simulink model "tracking"  (R2021a)
settings: Solver=ode45  StartTime=16665.7001  StopTime=33331.4002  MaxStep=0.1  RelTol=1e-8  AbsTol=1e-8
values from neighbouring files (symbols this model uses):
  spacecraft = struct()    [setup.m]
undefined symbols (not defined in the file or in its folder): actuators, constants, control, orbit
libraries: vrlib x6, library x3
settings Model: SimulationMode=accelerator  Creator=loren  LastModifiedBy=loren
settings SolverCC: ZeroCrossAlgorithm=Adaptive
settings DebuggingCC: IgnoredZcDiagnostic=none

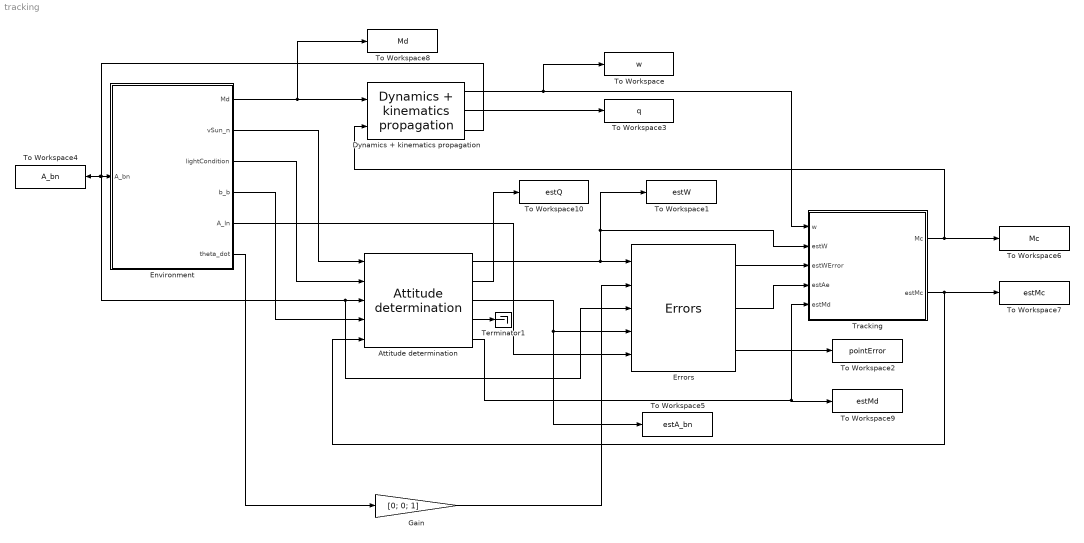
== system tracking ==
  Attitude determination : library/Attitude determination  SystemSampleTime=-1  VariantActivationTime=update diagram  Latency=0  AutoFrameSizeCalculation=off
  Dynamics + kinematics propagation : library/Dynamics + kinematics propagation  SystemSampleTime=-1  VariantActivationTime=update diagram  Latency=0  AutoFrameSizeCalculation=off
  Environment : Subsystem  AncestorBlock=library/Environment
  Errors : library/Errors  SystemSampleTime=-1  VariantActivationTime=update diagram  Latency=0  AutoFrameSizeCalculation=off
  Gain : Gain  Gain=[0; 0; 1]
  Terminator1 : Terminator
  To Workspace : ToWorkspace  VariableName=w  SampleTime=-1
  To Workspace1 : ToWorkspace  VariableName=estW  SampleTime=-1
  To Workspace10 : ToWorkspace  VariableName=estQ  SampleTime=-1
  To Workspace2 : ToWorkspace  VariableName=pointError  SampleTime=-1
  To Workspace3 : ToWorkspace  VariableName=q  SampleTime=-1
  To Workspace4 : ToWorkspace  VariableName=A_bn  SampleTime=-1
  To Workspace5 : ToWorkspace  VariableName=estA_bn  SampleTime=-1
  To Workspace6 : ToWorkspace  VariableName=Mc  SampleTime=-1
  To Workspace7 : ToWorkspace  VariableName=estMc  SampleTime=-1
  To Workspace8 : ToWorkspace  VariableName=Md  SampleTime=-1
  To Workspace9 : ToWorkspace  VariableName=estMd  SampleTime=-1
  Tracking : Subsystem  AncestorBlock=library/Tracking
  wires:
  Environment/5(A_ln) -> Errors/5
  Gain/1 -> Errors/2
  Dynamics + kinematics propagation/1 -> Tracking/1(w), To Workspace/1
  Errors/3 -> To Workspace2/1
  Environment/1(Md) -> To Workspace8/1, Dynamics + kinematics propagation/1
  Errors/1 -> Tracking/3(estWError)
  Tracking/2(estMc) -> Attitude determination/5, To Workspace7/1
  Errors/2 -> Tracking/4(estAe)
  Dynamics + kinematics propagation/2 -> To Workspace3/1
  Attitude determination/1 -> Tracking/2(estW), To Workspace1/1, Errors/1
  Environment/4(b_b) -> Attitude determination/4
  Attitude determination/2 -> To Workspace10/1
  Environment/6(theta_dot) -> Gain/1
  Dynamics + kinematics propagation/3 -> To Workspace4/1, Environment/1(A_bn), Errors/3, Attitude determination/3
  Environment/2(vSun_n) -> Attitude determination/1
  Tracking/1(Mc) -> Dynamics + kinematics propagation/2, To Workspace6/1
  Attitude determination/5 -> Tracking/5(estMd), To Workspace9/1
  Attitude determination/3 -> To Workspace5/1, Errors/4
  Environment/3(lightCondition) -> Attitude determination/2
  Attitude determination/4 -> Terminator1/1

== system tracking/Environment ==
  A_bn : Inport
  Disturbances : Subsystem
  Orbit propagator : Subsystem
  Md : Outport
  vSun_n : Outport  Port=2
  lightCondition : Outport  Port=3
  b_b : Outport  Port=4
  A_ln : Outport  Port=5
  theta_dot : Outport  Port=6
  wires:
  Orbit propagator/4(A_ln) -> A_ln/1
  Orbit propagator/5(theta_dot) -> theta_dot/1
  Disturbances/4(b_b) -> b_b/1
  Disturbances/3(lightCondition) -> lightCondition/1
  Disturbances/2(vSun_n) -> vSun_n/1
  Disturbances/1(Md) -> Md/1
  Orbit propagator/3(A_bl) -> Disturbances/4(A_bl)
  Orbit propagator/2(vvSc_n) -> Disturbances/3(vvSc_n)
  Orbit propagator/1(rrSc_n) -> Disturbances/2(rrSc_n)
  A_bn/1 -> Disturbances/1(A_bn), Orbit propagator/1(A_bn)

== system tracking/Tracking ==
  w : Inport
  estW : Inport  Port=2
  estWError : Inport  Port=3
  estAe : Inport  Port=4
  estMd : Inport  Port=5
  Ideal control law : Subsystem
  Reaction wheels : Subsystem  AncestorBlock=library/Reaction wheels
  Mc : Outport
  estMc : Outport  Port=2
  wires:
  Reaction wheels/2(estMc_RW) -> estMc/1
  Reaction wheels/1(Mc_RW) -> Mc/1
  estMd/1 -> Ideal control law/4(estMd)
  estAe/1 -> Ideal control law/3(estAe)
  estWError/1 -> Ideal control law/2(estWError)
  estW/1 -> Ideal control law/1(estW), Reaction wheels/3(estW)
  Ideal control law/1(Mc_id) -> Reaction wheels/1(targetMc)
  w/1 -> Reaction wheels/2(w)

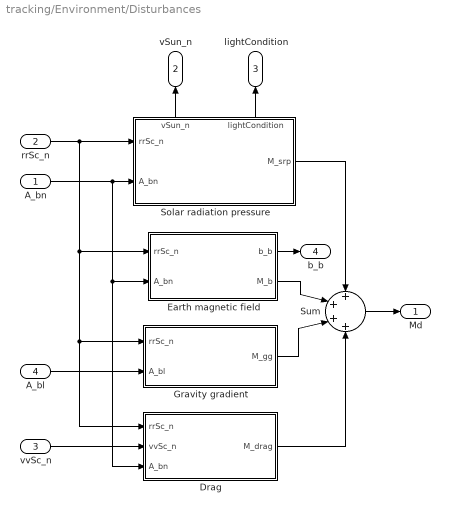
== system tracking/Environment/Disturbances ==
  A_bn : Inport
  rrSc_n : Inport  Port=2
  vvSc_n : Inport  Port=3
  A_bl : Inport  Port=4
  Drag : Subsystem
  Earth magnetic field : Subsystem
  Gravity gradient : Subsystem
  Solar radiation pressure : Subsystem
      settings: PortSchema="{\"entries\":[{\"content\":{\"sides\":[{\"content\":{\"connectorIds\":[\"In1\",\"In2\"]},\"type\":\"ConnectorPlacement.EquallySpacedRectSide\",\"uuid\":\"1c58e148-737e-4c26-8467-bf4a1427bac3\"},{\"content\":{\"connectorIds\":[\"Out1\"],\"side\":\"RIGHT\"},\"type\":\"ConnectorPlacement.EquallySpacedRectSide\",\"uuid\":\"1132a1c1-392d-4550-8b40-4ae647f3a6c1\"},{\"content\":{\"connectorIds\":[\"Out2\",\"Out3\"],\"side\":\"TOP\"},\"type\":\"ConnectorPlacement.EquallySpacedRectSide\",\"uuid\":\"8cec875a-7b2b-408d-843f-f50e353248f2\"},{\"content\":{\"connectorIds\":[],\"side\":\"HIDDEN\"},\"type\":\"ConnectorPlacement.EquallySpacedRectSide\",\"uuid\":\"95559ba3-4215-4144-a5e7-008848b1ca72\"}]},\"type\":\"ConnectorPlacement.EquallySpacedConnector\",\"uuid\":\"cb15f690-b6d7-424c-84c7-df23a46a4e4f\"}],\"packageUris\":[\"http://schema.mathworks.com/mf0/Connector/R2020b\"],\"version\":\"1.0\"}"
  Sum : Sum  Inputs=++++
  Md : Outport
  vSun_n : Outport  Port=2
  lightCondition : Outport  Port=3
  b_b : Outport  Port=4
  wires:
  Earth magnetic field/1(b_b) -> b_b/1
  Solar radiation pressure/3(lightCondition) -> lightCondition/1
  Solar radiation pressure/2(vSun_n) -> vSun_n/1
  A_bl/1 -> Gravity gradient/2(A_bl)
  Sum/1 -> Md/1
  Earth magnetic field/2(M_b) -> Sum/2
  Drag/1(M_drag) -> Sum/4
  Gravity gradient/1(M_gg) -> Sum/3
  rrSc_n/1 -> Solar radiation pressure/1(rrSc_n), Earth magnetic field/1(rrSc_n), Drag/1(rrSc_n), Gravity gradient/1(rrSc_n)
  vvSc_n/1 -> Drag/2(vvSc_n)
  A_bn/1 -> Earth magnetic field/2(A_bn), Drag/3(A_bn), Solar radiation pressure/2(A_bn)
  Solar radiation pressure/1(M_srp) -> Sum/1

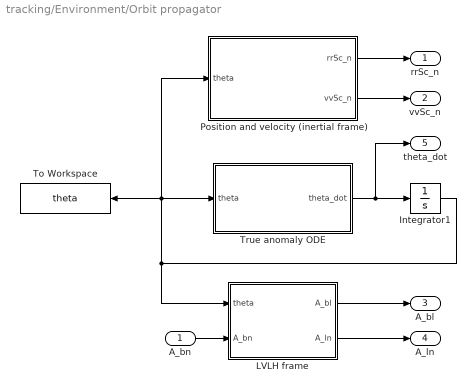
== system tracking/Environment/Orbit propagator ==
  A_bn : Inport
  Integrator1 : Integrator  InitialCondition=orbit.theta0
  LVLH frame : Subsystem
  Position and velocity (inertial frame) : Subsystem
  To Workspace : ToWorkspace  VariableName=theta  SampleTime=-1
  True anomaly ODE : Subsystem
  rrSc_n : Outport
  vvSc_n : Outport  Port=2
  A_bl : Outport  Port=3
  A_ln : Outport  Port=4
  theta_dot : Outport  Port=5
  wires:
  LVLH frame/2(A_ln) -> A_ln/1
  A_bn/1 -> LVLH frame/2(A_bn)
  LVLH frame/1(A_bl) -> A_bl/1
  Position and velocity (inertial frame)/2(vvSc_n) -> vvSc_n/1
  Position and velocity (inertial frame)/1(rrSc_n) -> rrSc_n/1
  Integrator1/1 -> To Workspace/1, Position and velocity (inertial frame)/1(theta), True anomaly ODE/1(theta), LVLH frame/1(theta)
  True anomaly ODE/1(theta_dot) -> theta_dot/1, Integrator1/1

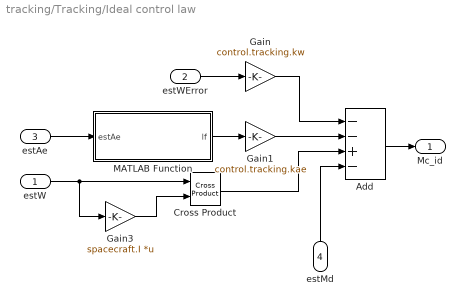
== system tracking/Tracking/Ideal control law ==
  estW : Inport
  estWError : Inport  Port=2
  estAe : Inport  Port=3
  estMd : Inport  Port=4
  Add : Sum  Inputs=--+-
  Cross Product : vrlib/Utilities/Cross Product
  Gain : Gain  Gain=control.tracking.kw
  Gain1 : Gain  Gain=control.tracking.kae
  Gain3 : Gain  Gain=spacecraft.I  Multiplication=Matrix(K*u) (u vector)
  MATLAB Function : MATLAB Function  TreatAsAtomicUnit=on
  Mc_id : Outport
  wires:
  Cross Product/1 -> Add/3
  estW/1 -> Cross Product/1, Gain3/1
  estWError/1 -> Gain/1
  Gain1/1 -> Add/2
  estMd/1 -> Add/4
  Gain3/1 -> Cross Product/2
  Gain/1 -> Add/1
  estAe/1 -> MATLAB Function/1(estAe)
  MATLAB Function/1(lf) -> Gain1/1
  Add/1 -> Mc_id/1

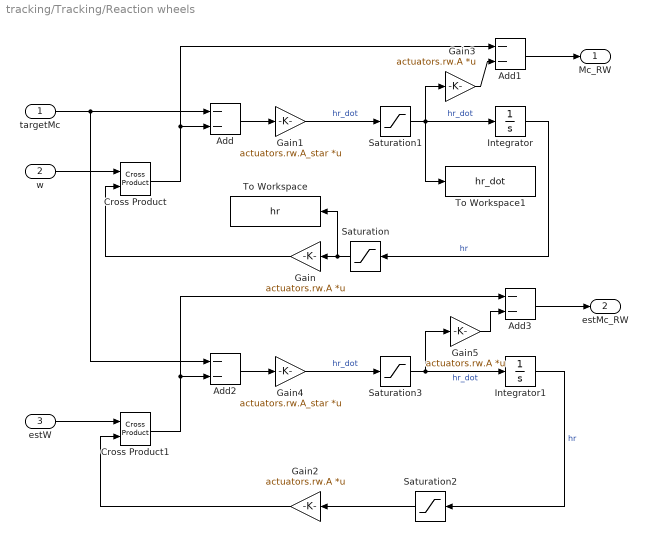
== system tracking/Tracking/Reaction wheels ==
  targetMc : Inport
  w : Inport  Port=2
  estW : Inport  Port=3
  Add{,1..3} (4 alike) : Sum  Inputs=--
  Cross Product : vrlib/Utilities/Cross Product
  Cross Product1 : vrlib/Utilities/Cross Product
  Gain{,2..3,5} (4 alike) : Gain  Gain=actuators.rw.A  Multiplication=Matrix(K*u) (u vector)
  Gain1 : Gain  Gain=actuators.rw.A_star  Multiplication=Matrix(K*u) (u vector)
  Gain4 : Gain  Gain=actuators.rw.A_star  Multiplication=Matrix(K*u) (u vector)
  Integrator : Integrator  InitialCondition=actuators.rw.hr0
  Integrator1 : Integrator  InitialCondition=actuators.rw.hr0
  Saturation : Saturate  UpperLimit=actuators.rw.h_max  LowerLimit=-actuators.rw.h_max
  Saturation1 : Saturate  UpperLimit=actuators.rw.hdot_max  LowerLimit=-actuators.rw.hdot_max
  Saturation2 : Saturate  UpperLimit=actuators.rw.h_max  LowerLimit=-actuators.rw.h_max
  Saturation3 : Saturate  UpperLimit=actuators.rw.hdot_max  LowerLimit=-actuators.rw.hdot_max
  To Workspace : ToWorkspace  VariableName=hr  SampleTime=-1
  To Workspace1 : ToWorkspace  VariableName=hr_dot  SampleTime=-1
  Mc_RW : Outport
  estMc_RW : Outport  Port=2
  wires:
  w/1 -> Cross Product/1
  Gain/1 -> Cross Product/2
  Cross Product/1 -> Add/2, Add1/1
  Gain1/1 -> Saturation1/1  "hr_dot"
  Integrator/1 -> Saturation/1  "hr"
  Saturation/1 -> To Workspace/1, Gain/1
  Add1/1 -> Mc_RW/1
  Add/1 -> Gain1/1
  Gain3/1 -> Add1/2
  Saturation1/1 -> To Workspace1/1, Gain3/1, Integrator/1  "hr_dot"
  Gain5/1 -> Add3/2
  Add3/1 -> estMc_RW/1
  Add2/1 -> Gain4/1
  Saturation3/1 -> Integrator1/1, Gain5/1  "hr_dot"
  Cross Product1/1 -> Add2/2, Add3/1
  Integrator1/1 -> Saturation2/1  "hr"
  estW/1 -> Cross Product1/1
  targetMc/1 -> Add2/1, Add/1
  Saturation2/1 -> Gain2/1
  Gain2/1 -> Cross Product1/2
  Gain4/1 -> Saturation3/1  "hr_dot"

== system tracking/Environment/Disturbances/Drag ==
  rrSc_n : Inport
  vvSc_n : Inport  Port=2
  A_bn : Inport  Port=3
  Constant : Constant  Value=constants.rho
  MATLAB Function : MATLAB Function  TreatAsAtomicUnit=on
  M_drag : Outport
  wires:
  Constant/1 -> MATLAB Function/4(rho)
  A_bn/1 -> MATLAB Function/3(A_bn)
  vvSc_n/1 -> MATLAB Function/2(vvSc_n)
  MATLAB Function/1(mDrag) -> M_drag/1
  rrSc_n/1 -> MATLAB Function/1(rrSc_n)

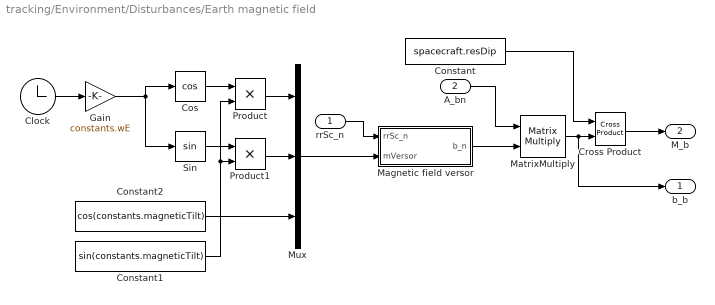
== system tracking/Environment/Disturbances/Earth magnetic field ==
  rrSc_n : Inport
  A_bn : Inport  Port=2
  Clock : Clock
  Constant : Constant  Value=spacecraft.resDip
  Constant1 : Constant  Value=sin(constants.magneticTilt)
  Constant2 : Constant  Value=cos(constants.magneticTilt)
  Cos : Trigonometry  Operator=cos
  Cross Product : vrlib/Utilities/Cross Product
  Gain : Gain  Gain=constants.wE
  Magnetic field versor : Subsystem
  MatrixMultiply : Product  Multiplication=Matrix(*)
  Mux : Mux  Inputs=3
  Product : Product
  Product1 : Product
  Sin : Trigonometry
  b_b : Outport
  M_b : Outport  Port=2
  wires:
  Cross Product/1 -> M_b/1
  MatrixMultiply/1 -> Cross Product/2, b_b/1
  Magnetic field versor/1(b_n) -> MatrixMultiply/2
  Mux/1 -> Magnetic field versor/2(mVersor)
  rrSc_n/1 -> Magnetic field versor/1(rrSc_n)
  A_bn/1 -> MatrixMultiply/1
  Constant1/1 -> Product1/2, Product/2
  Product1/1 -> Mux/2
  Product/1 -> Mux/1
  Cos/1 -> Product/1
  Sin/1 -> Product1/1
  Constant2/1 -> Mux/3
  Gain/1 -> Cos/1, Sin/1
  Constant/1 -> Cross Product/1
  Clock/1 -> Gain/1

== system tracking/Environment/Disturbances/Gravity gradient ==
  rrSc_n : Inport
  A_bl : Inport  Port=2
  Constant : Constant  Value=[1 0 0]
  Gravity gradient : Subsystem
  MatrixMultiply : Product  Multiplication=Matrix(*)
  M_gg : Outport
  wires:
  rrSc_n/1 -> Gravity gradient/1(rrSc_n)
  Gravity gradient/1(M_gg) -> M_gg/1
  A_bl/1 -> MatrixMultiply/1
  MatrixMultiply/1 -> Gravity gradient/2(c)  "c"
  Constant/1 -> MatrixMultiply/2

== system tracking/Environment/Disturbances/Solar radiation pressure ==
  note: Determine whether the s/c is in sunlight or not
  rrSc_n : Inport
  A_bn : Inport  Port=2
  If : If  IfExpression=u1 == 1
  Merge : Merge
  SRP: active : Subsystem  TreatAsAtomicUnit=on
  SRP: non-active : Subsystem  TreatAsAtomicUnit=on
  Shadow cone of the Earth : Subsystem
  Sun position in the Earth inertial frame : Subsystem
  M_srp : Outport
  vSun_n : Outport  Port=2
  lightCondition : Outport  Port=3
  wires:
  A_bn/1 -> SRP: active/3(A_bn)
  SRP: active/2(vSun_n) -> vSun_n/1
  Sun position in the Earth inertial frame/1(rrSun_n) -> Shadow cone of the Earth/2(rrSun_n), SRP: active/2(rrSun_n)
  SRP: active/1(mSRP) -> Merge/1
  Merge/1 -> M_srp/1
  rrSc_n/1 -> Shadow cone of the Earth/1(rrSc_n), SRP: active/1(rrSc_n)
  SRP: non-active/1(mSRP) -> Merge/2
  If/1 -> SRP: active/Action
  If/2 -> SRP: non-active/Action
  Shadow cone of the Earth/1(lightCondition) -> If/1, lightCondition/1

== system tracking/Environment/Orbit propagator/LVLH frame ==
  theta : Inport
  A_bn : Inport  Port=2
  LVLH to inclined orbit frame : Subsystem
  Product : Product  Multiplication=Matrix(*)
  Product1 : Product  Multiplication=Matrix(*)
  R1(i) : Constant  Value=[1 0 0; 0 cos(orbit.i) sin(orbit.i); 0 -sin(orbit.i) cos(orbit.i)];
  Transpose : Math  Operator=transpose  SaturateOnIntegerOverflow=on
  A_bl : Outport
  A_ln : Outport  Port=2
  wires:
  LVLH to inclined orbit frame/1(A_li) -> Product/1
  theta/1 -> LVLH to inclined orbit frame/1(theta)
  R1(i)/1 -> Product/2
  Product1/1 -> A_bl/1  "A_bl"
  A_bn/1 -> Product1/1
  Product/1 -> Transpose/1, A_ln/1
  Transpose/1 -> Product1/2  "A_nl"

== system tracking/Environment/Orbit propagator/Position and velocity (inertial frame) ==
  theta : Inport
  Matrix Multiply : Product  Multiplication=Matrix(*)
  Matrix Multiply1 : Product  Multiplication=Matrix(*)
  Position and velocity (perifocal frame) : Subsystem
  R1(i) : Constant  Value=[1 0 0; 0 cos(orbit.i) sin(orbit.i); 0 -sin(orbit.i) cos(orbit.i)];
  R3(OM) : Constant  Value=[cos(orbit.OM), sin(orbit.OM), 0; -sin(orbit.OM), cos(orbit.OM), 0; 0, 0, 1]
  R3(om) : Constant  Value=[cos(orbit.om), sin(orbit.om), 0; -sin(orbit.om), cos(orbit.om), 0; 0, 0, 1]
  Rotation matrix (perifocal-inertial) : Product  Inputs=3  Multiplication=Matrix(*)
  Transpose : Math  Operator=transpose  SaturateOnIntegerOverflow=on
  rrSc_n : Outport
  vvSc_n : Outport  Port=2
  wires:
  theta/1 -> Position and velocity (perifocal frame)/1(theta)
  Position and velocity (perifocal frame)/1(rrSc_pf) -> Matrix Multiply/2
  R3(OM)/1 -> Rotation matrix (perifocal-inertial)/3
  Transpose/1 -> Matrix Multiply/1, Matrix Multiply1/1
  Rotation matrix (perifocal-inertial)/1 -> Transpose/1
  R1(i)/1 -> Rotation matrix (perifocal-inertial)/2
  R3(om)/1 -> Rotation matrix (perifocal-inertial)/1
  Matrix Multiply1/1 -> vvSc_n/1
  Position and velocity (perifocal frame)/2(vvSc_pf) -> Matrix Multiply1/2
  Matrix Multiply/1 -> rrSc_n/1

== system tracking/Environment/Orbit propagator/True anomaly ODE ==
  theta : Inport
  Add : Sum
  Constant1 : Constant
  Cos : Trigonometry  Operator=cos
  Gain : Gain  Gain=sqrt(constants.mu/orbit.a^3)
  Gain1 : Gain  Gain=(1 - orbit.e^2)^(-3/2)
  Gain2 : Gain  Gain=orbit.e
  Power : Math  Operator=square  SaturateOnIntegerOverflow=on
  theta_dot : Outport
  wires:
  Gain1/1 -> theta_dot/1
  Gain/1 -> Gain1/1
  Power/1 -> Gain/1
  Add/1 -> Power/1
  Gain2/1 -> Add/2
  Cos/1 -> Gain2/1
  Constant1/1 -> Add/1
  theta/1 -> Cos/1

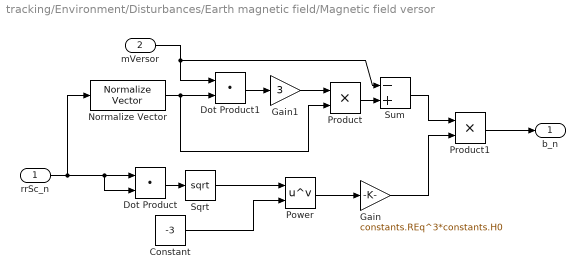
== system tracking/Environment/Disturbances/Earth magnetic field/Magnetic field versor ==
  rrSc_n : Inport
  mVersor : Inport  Port=2
  Constant : Constant  Value=-3
  Dot Product : DotProduct  InputSameDT=on  OutDataTypeStr=Inherit: Inherit via internal rule
  Dot Product1 : DotProduct  InputSameDT=on  OutDataTypeStr=Inherit: Inherit via internal rule
  Gain : Gain  Gain=constants.REq^3*constants.H0
  Gain1 : Gain  Gain=3
  Normalize Vector : vrlib/Utilities/Normalize Vector  maxzero=0
  Power : Math  Operator=pow  SaturateOnIntegerOverflow=on
  Product : Product
  Product1 : Product
  Sqrt : Sqrt  SaturateOnIntegerOverflow=on
  Sum : Sum  Inputs=-+
  b_n : Outport
  wires:
  Product1/1 -> b_n/1
  Gain/1 -> Product1/2
  Sum/1 -> Product1/1
  Product/1 -> Sum/2
  Gain1/1 -> Product/1
  Dot Product1/1 -> Gain1/1
  mVersor/1 -> Dot Product1/1, Sum/1
  Normalize Vector/1 -> Dot Product1/2, Product/2
  Power/1 -> Gain/1
  Sqrt/1 -> Power/1
  Dot Product/1 -> Sqrt/1
  Constant/1 -> Power/2
  rrSc_n/1 -> Dot Product/1, Dot Product/2, Normalize Vector/1

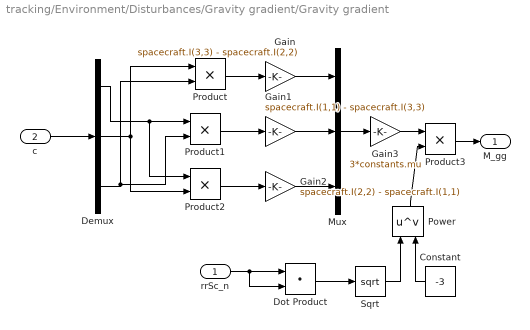
== system tracking/Environment/Disturbances/Gravity gradient/Gravity gradient ==
  rrSc_n : Inport
  c : Inport  Port=2
  Constant : Constant  Value=-3
  Demux : Demux  Outputs=3
  Dot Product : DotProduct  InputSameDT=on  OutDataTypeStr=Inherit: Inherit via internal rule
  Gain : Gain  Gain=spacecraft.I(3,3) - spacecraft.I(2,2)
  Gain1 : Gain  Gain=spacecraft.I(1,1) - spacecraft.I(3,3)
  Gain2 : Gain  Gain=spacecraft.I(2,2) - spacecraft.I(1,1)
  Gain3 : Gain  Gain=3*constants.mu
  Mux : Mux  Inputs=3
  Power : Math  Operator=pow  SaturateOnIntegerOverflow=on
  Product{,1..3} (4 alike) : Product
  Sqrt : Sqrt  SaturateOnIntegerOverflow=on
  M_gg : Outport
  wires:
  Constant/1 -> Power/2
  Power/1 -> Product3/2
  Sqrt/1 -> Power/1
  Dot Product/1 -> Sqrt/1
  rrSc_n/1 -> Dot Product/1, Dot Product/2
  Product3/1 -> M_gg/1
  Gain3/1 -> Product3/1
  Mux/1 -> Gain3/1
  Gain/1 -> Mux/1
  Gain1/1 -> Mux/2
  Gain2/1 -> Mux/3
  Demux/1 -> Product1/1, Product2/1
  Demux/3 -> Product/2, Product1/2
  Demux/2 -> Product/1, Product2/2
  Product2/1 -> Gain2/1
  Product1/1 -> Gain1/1
  Product/1 -> Gain/1
  c/1 -> Demux/1

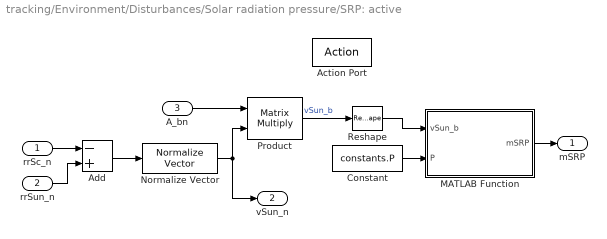
== system tracking/Environment/Disturbances/Solar radiation pressure/SRP: active ==
  rrSc_n : Inport
  rrSun_n : Inport  Port=2
  A_bn : Inport  Port=3
  Action Port : ActionPort  ActionPortLabel=if(u1 == 1)
  Add : Sum  Inputs=-+
  Constant : Constant  Value=constants.P
  MATLAB Function : MATLAB Function  TreatAsAtomicUnit=on
  Normalize Vector : vrlib/Utilities/Normalize Vector  maxzero=0
  Product : Product  Multiplication=Matrix(*)
  Reshape : Reshape  OutputDimensionality=Column vector (2-D)
  mSRP : Outport
  vSun_n : Outport  Port=2
  wires:
  Reshape/1 -> MATLAB Function/1(vSun_b)
  Constant/1 -> MATLAB Function/2(P)
  rrSc_n/1 -> Add/1
  MATLAB Function/1(mSRP) -> mSRP/1
  Add/1 -> Normalize Vector/1
  Normalize Vector/1 -> Product/2, vSun_n/1
  Product/1 -> Reshape/1  "vSun_b"
  rrSun_n/1 -> Add/2
  A_bn/1 -> Product/1

== system tracking/Environment/Disturbances/Solar radiation pressure/SRP: non-active ==
  Action Port : ActionPort  ActionPortLabel=else
  Constant1 : Constant  Value=[0;0;0]
  mSRP : Outport
  wires:
  Constant1/1 -> mSRP/1

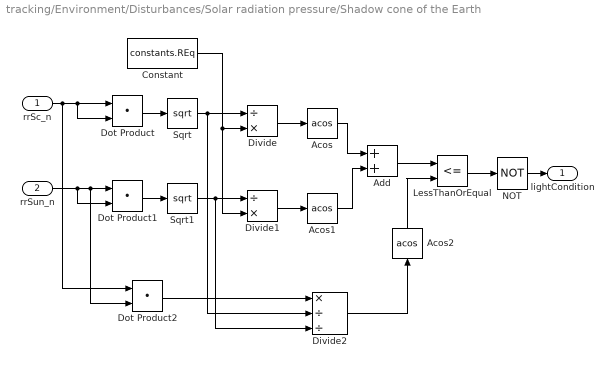
== system tracking/Environment/Disturbances/Solar radiation pressure/Shadow cone of the Earth ==
  rrSc_n : Inport
  rrSun_n : Inport  Port=2
  Acos : Trigonometry  Operator=acos
  Acos1 : Trigonometry  Operator=acos
  Acos2 : Trigonometry  Operator=acos
  Add : Sum
  Constant : Constant  Value=constants.REq
  Divide : Product  Inputs=/*
  Divide1 : Product  Inputs=/*
  Divide2 : Product  Inputs=*//
  Dot Product : DotProduct  InputSameDT=on  OutDataTypeStr=Inherit: Inherit via internal rule
  Dot Product1 : DotProduct  InputSameDT=on  OutDataTypeStr=Inherit: Inherit via internal rule
  Dot Product2 : DotProduct  InputSameDT=on  OutDataTypeStr=Inherit: Inherit via internal rule
  LessThanOrEqual : RelationalOperator  Operator=<=  OutDataTypeStr=boolean  RndMeth=Simplest
  NOT : Logic  Operator=NOT  IconShape=distinctive  AllPortsSameDT=off  OutDataTypeStr=boolean
  Sqrt : Sqrt  SaturateOnIntegerOverflow=on
  Sqrt1 : Sqrt  SaturateOnIntegerOverflow=on
  lightCondition : Outport
  wires:
  Acos2/1 -> LessThanOrEqual/2
  NOT/1 -> lightCondition/1
  LessThanOrEqual/1 -> NOT/1
  Divide2/1 -> Acos2/1
  Add/1 -> LessThanOrEqual/1
  Acos1/1 -> Add/2
  Acos/1 -> Add/1
  Dot Product2/1 -> Divide2/1
  Divide1/1 -> Acos1/1
  Divide/1 -> Acos/1
  Constant/1 -> Divide/2, Divide1/2
  Sqrt1/1 -> Divide1/1, Divide2/3
  Sqrt/1 -> Divide/1, Divide2/2
  rrSun_n/1 -> Dot Product1/1, Dot Product2/2, Dot Product1/2
  Dot Product1/1 -> Sqrt1/1
  Dot Product/1 -> Sqrt/1
  rrSc_n/1 -> Dot Product/1, Dot Product/2, Dot Product2/1

== system tracking/Environment/Disturbances/Solar radiation pressure/Sun position in the Earth inertial frame ==
  Clock : Clock
  Cos : Trigonometry  Operator=cos
  Gain : Gain  Gain=constants.nSun
  Gain1 : Gain  Gain=cos(constants.oblAngle)
  Gain2 : Gain  Gain=sin(constants.oblAngle)
  Gain3 : Gain  Gain=1*constants.AU
  Mux : Mux  Inputs=3
  Sin1 : Trigonometry
  rrSun_n : Outport
  wires:
  Gain3/1 -> rrSun_n/1
  Cos/1 -> Mux/1
  Sin1/1 -> Gain1/1, Gain2/1
  Mux/1 -> Gain3/1
  Gain1/1 -> Mux/2
  Gain/1 -> Cos/1, Sin1/1
  Clock/1 -> Gain/1
  Gain2/1 -> Mux/3

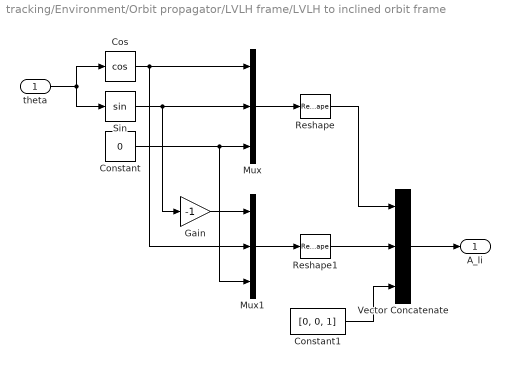
== system tracking/Environment/Orbit propagator/LVLH frame/LVLH to inclined orbit frame ==
  theta : Inport
  Constant : Constant  Value=0
  Constant1 : Constant  Value=[0, 0, 1]  VectorParams1D=off
  Cos : Trigonometry  Operator=cos
  Gain : Gain  Gain=-1
  Mux : Mux  Inputs=3
  Mux1 : Mux  Inputs=3
  Reshape : Reshape  OutputDimensionality=Row vector (2-D)
  Reshape1 : Reshape  OutputDimensionality=Row vector (2-D)
  Sin : Trigonometry
  Vector Concatenate : Concatenate  NumInputs=3  Mode=Multidimensional array
  A_li : Outport
  wires:
  Reshape1/1 -> Vector Concatenate/2
  Reshape/1 -> Vector Concatenate/1
  Vector Concatenate/1 -> A_li/1
  Mux1/1 -> Reshape1/1
  Constant1/1 -> Vector Concatenate/3
  Mux/1 -> Reshape/1
  Gain/1 -> Mux1/1
  Constant/1 -> Mux/3, Mux1/3
  Sin/1 -> Mux/2, Gain/1
  Cos/1 -> Mux/1, Mux1/2
  theta/1 -> Cos/1, Sin/1

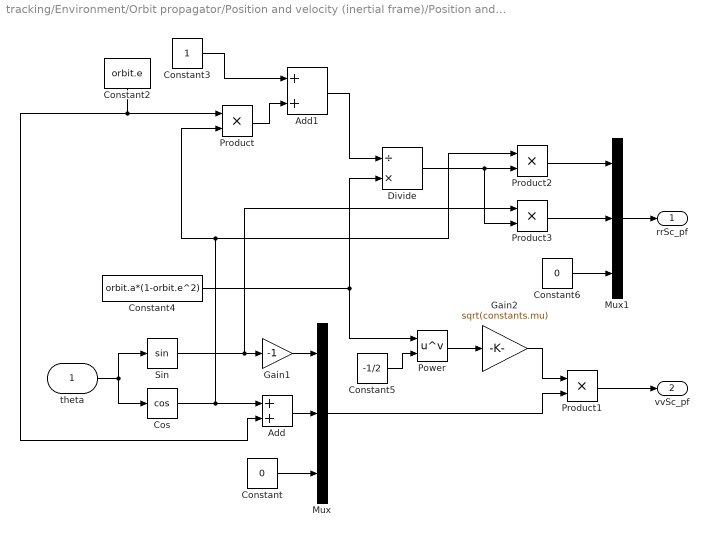
== system tracking/Environment/Orbit propagator/Position and velocity (inertial frame)/Position and velocity (perifocal frame) ==
  theta : Inport
  Add : Sum
  Add1 : Sum
  Constant : Constant  Value=0
  Constant2 : Constant  Value=orbit.e
  Constant3 : Constant
  Constant4 : Constant  Value=orbit.a*(1-orbit.e^2)
  Constant5 : Constant  Value=-1/2
  Constant6 : Constant  Value=0
  Cos : Trigonometry  Operator=cos
  Divide : Product  Inputs=/*
  Gain1 : Gain  Gain=-1
  Gain2 : Gain  Gain=sqrt(constants.mu)
  Mux : Mux  Inputs=3
  Mux1 : Mux  Inputs=3
  Power : Math  Operator=pow  SaturateOnIntegerOverflow=on
  Product{,1..3} (4 alike) : Product
  Sin : Trigonometry
  rrSc_pf : Outport
  vvSc_pf : Outport  Port=2
  wires:
  Mux1/1 -> rrSc_pf/1
  Constant6/1 -> Mux1/3
  Product3/1 -> Mux1/2
  Product2/1 -> Mux1/1
  Divide/1 -> Product2/2, Product3/2
  Gain2/1 -> Product1/1
  Power/1 -> Gain2/1
  Constant5/1 -> Power/2
  Constant4/1 -> Power/1, Divide/2
  Add1/1 -> Divide/1
  Product/1 -> Add1/2
  Constant2/1 -> Product/1, Add/2
  Constant3/1 -> Add1/1
  Product1/1 -> vvSc_pf/1
  Constant/1 -> Mux/3
  Add/1 -> Mux/2
  Gain1/1 -> Mux/1
  Cos/1 -> Add/1, Product/2, Product2/1
  Sin/1 -> Gain1/1, Product3/1
  Mux/1 -> Product1/2
  theta/1 -> Sin/1, Cos/1

== matlab function tracking/Environment/Disturbances/Solar radiation pressure/SRP: active/MATLAB Function ==
  data: vSun_b input; P input; mSRP output; surfaces parameter
function mSRP = srp(vSun_b, P, surfaces)

rSurf = surfaces.rSurf;
n = surfaces.n;
A = surfaces.A;
rhoS = surfaces.rhoS;
rhoD = surfaces.rhoD;

% Preallocation
mSRP = zeros(3,1);

% Loop on the number of surfaces
for k = 1:size(rSurf,1)
    % Extraction of the normal vector
    n_b = n(:,k);
    s_dot = dot(vSun_b, n_b);
    if s_dot > 0
        rhoS_temp = rhoS(k);
        Fsrp_i = - P*A(k)*s_dot.*((1-rhoS_temp).*vSun_b +...
            (2*rhoS_temp*s_dot + 2/3*rhoD(k)).*n_b);
        mSRP = mSRP + cross(rSurf(:,k), Fsrp_i);
    end
end

end

== matlab function tracking/Environment/Disturbances/Drag/MATLAB Function ==
  data: rrSc_n input; mDrag output; vvSc_n input; A_bn input; rho input; surfaces parameter
function  mDrag = drag(rrSc_n, vvSc_n, A_bn, rho, surfaces)

rSurf = surfaces.rSurf;
n = surfaces.n;
A = surfaces.A;
cd = surfaces.cd;

% Earth's angular speed
wE = 7.2921150e-5; %[rad/s]
% Relative velocity of the s/c with respect to the atmosphere
vvRel_n = [vvSc_n(1) + wE*rrSc_n(2); vvSc_n(2) - wE*rrSc_n(1); vvSc_n(3)]*1e3;
vvRel_b = A_bn*vvRel_n;

vRel_b = norm(vvRel_b);
vvVersor = vvRel_b/vRel_b;

c = -1/2*rho*cd*vRel_b^2.*vvVersor;

mDrag = zeros(3,1);

for k = 1:size(rSurf,1)
    % Extracting the normal unit vector
    n_dot = dot(n(:,k), vvVersor);
    if n_dot > 0
        A_cross = A(k)*n_dot;
        Fdrag_i = c*A_cross;
        mDrag = mDrag + cross(rSurf(:,k), Fdrag_i);
    end
end

end

== matlab function tracking/Tracking/Ideal control law/MATLAB Function ==
  data: estAe input; lf output
function lf = linearFunction(estAe)

lf = [estAe(2,3) - estAe(3,2);...
    estAe(3,1) - estAe(1,3);...
    estAe(1,2) - estAe(2,1)];

end
